simulink model "pendulum_sim"  (R2019b)
settings: Solver=VariableStepAuto  StartTime=0.0  StopTime=40  RelTol=1e-3
values from neighbouring files (symbols this model uses):
  A = 1.15    [pendulum_solution_prac.m]
  C = 5    [pendulum_solution_prac.m]
  W = 0.6666    [pendulum_solution_prac.m]
  x0 = [0.5;0.2]    [pendulum_solution_prac.m]
  x0_pert = [0.52;0.23]    [pendulum_solution_prac.m]
undefined symbols (not defined in the file or in its folder): pendulum
libraries: simulink x1
settings Model: Creator=user  LastModifiedBy=user

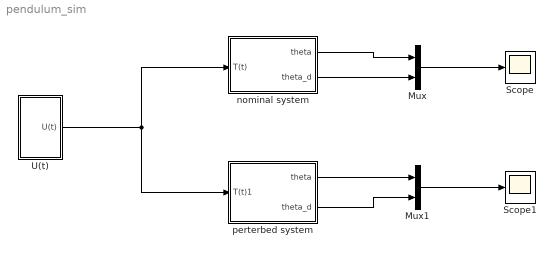
== system pendulum_sim ==
  Mux : Mux  Inputs=2
  Mux1 : Mux  Inputs=2
  Scope : Scope
  Scope1 : Scope
  U(t) : Subsystem
  nominal system : Subsystem
  perterbed system : Subsystem
  wires:
  U(t)/1(U(t)) -> nominal system/1(T(t)), perterbed system/1(T(t)1)
  nominal system/1(theta) -> Mux/1
  nominal system/2(theta_d) -> Mux/2
  perterbed system/2(theta_d) -> Mux1/2
  perterbed system/1(theta) -> Mux1/1
  Mux/1 -> Scope/1
  Mux1/1 -> Scope1/1

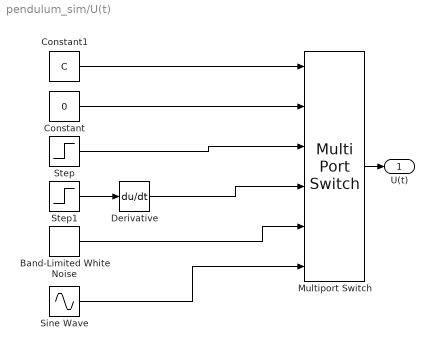
== system pendulum_sim/U(t) ==
  Band-Limited White Noise : simulink/Sources/Band-Limited White Noise  Cov=[0.1]  Ts=1  seed=[23341]
  Constant : Constant  Value=0
  Constant1 : Constant  Value=C
  Derivative : Derivative
  Multiport Switch : MultiPortSwitch  Inputs=5
  Sine Wave : Sin  Amplitude=A  Frequency=W  SampleTime=0
  Step : Step  Time=0  After=20  SampleTime=0
  Step1 : Step  Time=0  After=20  SampleTime=0
  U(t) : Outport
  wires:
  Step/1 -> Multiport Switch/3
  Sine Wave/1 -> Multiport Switch/6
  Band-Limited White Noise/1 -> Multiport Switch/5
  Step1/1 -> Derivative/1
  Multiport Switch/1 -> U(t)/1
  Constant/1 -> Multiport Switch/2
  Derivative/1 -> Multiport Switch/4
  Constant1/1 -> Multiport Switch/1

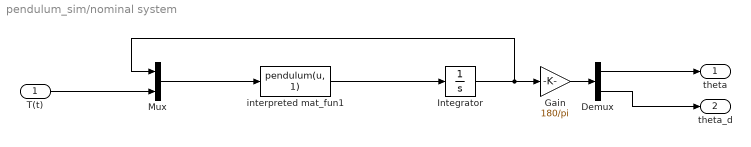
== system pendulum_sim/nominal system ==
  T(t) : Inport
  Demux : Demux  Outputs=2
  Gain : Gain  Gain=180/pi
  Integrator : Integrator  InitialCondition=x0
  Mux : Mux  Inputs=2
  interpreted mat_fun1 : MATLABFcn  MATLABFcn=pendulum(u, 1)
  theta : Outport
  theta_d : Outport  Port=2
  wires:
  Demux/2 -> theta_d/1
  Integrator/1 -> Mux/1, Gain/1
  Mux/1 -> interpreted mat_fun1/1
  T(t)/1 -> Mux/2
  Demux/1 -> theta/1
  interpreted mat_fun1/1 -> Integrator/1
  Gain/1 -> Demux/1

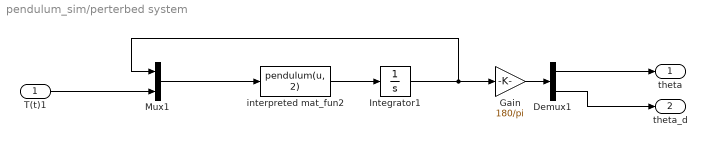
== system pendulum_sim/perterbed system ==
  T(t)1 : Inport
  Demux1 : Demux  Outputs=2
  Gain : Gain  Gain=180/pi
  Integrator1 : Integrator  InitialCondition=x0_pert
  Mux1 : Mux  Inputs=2
  interpreted mat_fun2 : MATLABFcn  MATLABFcn=pendulum(u, 2)
  theta : Outport
  theta_d : Outport  Port=2
  wires:
  Demux1/2 -> theta_d/1
  Demux1/1 -> theta/1
  T(t)1/1 -> Mux1/2
  Mux1/1 -> interpreted mat_fun2/1
  interpreted mat_fun2/1 -> Integrator1/1
  Integrator1/1 -> Mux1/1, Gain/1
  Gain/1 -> Demux1/1
